simulink subsystem "A_LN_elliptical_inclined"  (R2022b)
settings: Solver=VariableStepAuto  StartTime=0.0  StopTime=10.0  RelTol=1e-3
undefined symbols (not defined in the file or in its folder): settings
libraries: matrix_library x1
settings Model: Creator=robertopistonenascone  LastModifiedBy=robertopistonenascone

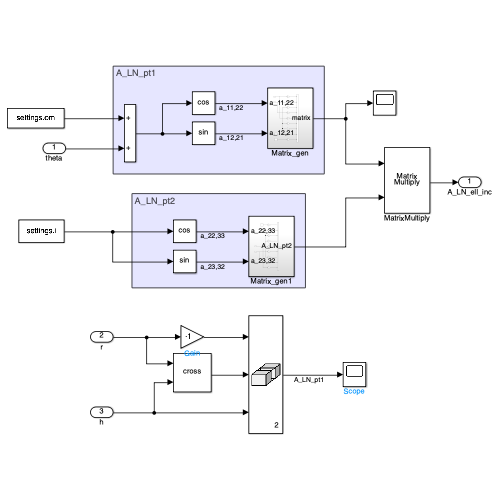
[thumbnail: Simulink's stored preview of the top-level diagram]
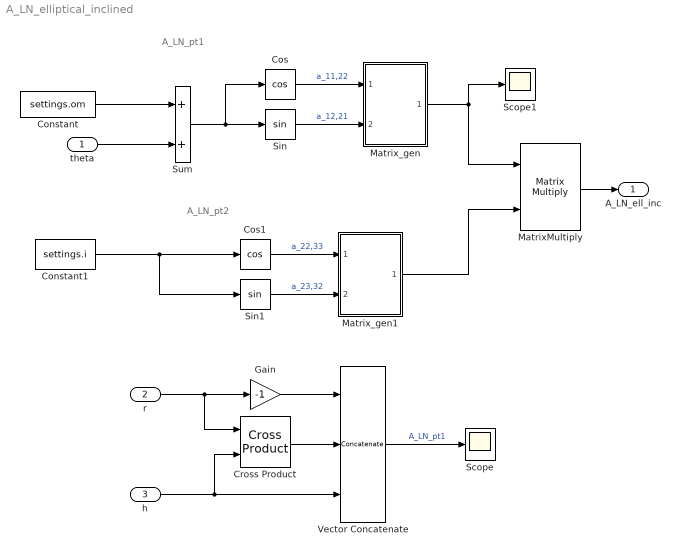
== system A_LN_elliptical_inclined ==
  note: A_LN_pt1
  note: A_LN_pt2
  theta : Inport
  r : Inport  Port=2
  h : Inport  Port=3
  Constant : Constant  Value=settings.om
  Constant1 : Constant  Value=settings.i
  Cos : Trigonometry  Operator=cos
  Cos1 : Trigonometry  Operator=cos
  Cross Product : matrix_library/Cross Product
  Gain : Gain  Gain=-1
  MatrixMultiply : Product  Multiplication=Matrix(*)
  Matrix_gen : Subsystem
  Matrix_gen1 : Subsystem
  Scope : Scope
  Scope1 : Scope
  Sin : Trigonometry
  Sin1 : Trigonometry
  Sum : Sum
  Vector Concatenate : Concatenate  NumInputs=3  Mode=Multidimensional array  ConcatenateDimension=2
  A_LN_ell_inc : Outport
  wires:
  MatrixMultiply/1 -> A_LN_ell_inc/1
  Matrix_gen/1(matrix) -> MatrixMultiply/1, Scope1/1
  Matrix_gen1/1(A_LN_pt2) -> MatrixMultiply/2
  Sum/1 -> Cos/1, Sin/1
  Cos1/1 -> Matrix_gen1/1(a_22,33)  "a_22,33"
  Constant1/1 -> Cos1/1, Sin1/1
  Cos/1 -> Matrix_gen/1(a_11,22)  "a_11,22"
  Sin/1 -> Matrix_gen/2(a_12,21)  "a_12,21"
  Constant/1 -> Sum/1
  Sin1/1 -> Matrix_gen1/2(a_23,32)  "a_23,32"
  theta/1 -> Sum/2
  Cross Product/1 -> Vector Concatenate/2
  r/1 -> Cross Product/1, Gain/1
  h/1 -> Cross Product/2, Vector Concatenate/3
  Vector Concatenate/1 -> Scope/1  "A_LN_pt1"
  Gain/1 -> Vector Concatenate/1

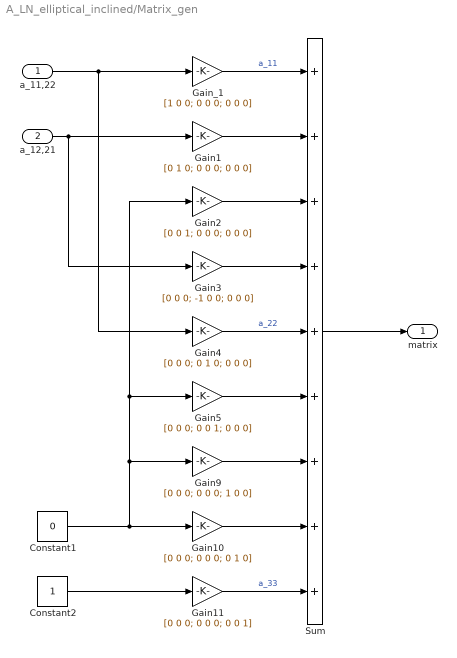
== system A_LN_elliptical_inclined/Matrix_gen ==
  a_11,22 : Inport
  a_12,21 : Inport  Port=2
  Constant1 : Constant  Value=0
  Constant2 : Constant
  Gain1 : Gain  Gain=[0 1 0; 0 0 0; 0 0 0]
  Gain10 : Gain  Gain=[0 0 0; 0 0 0; 0 1 0]
  Gain11 : Gain  Gain=[0 0 0; 0 0 0; 0 0 1]
  Gain2 : Gain  Gain=[0 0 1; 0 0 0; 0 0 0]
  Gain3 : Gain  Gain=[0 0 0; -1 0 0; 0 0 0]
  Gain4 : Gain  Gain=[0 0 0; 0 1 0; 0 0 0]
  Gain5 : Gain  Gain=[0 0 0; 0 0 1; 0 0 0]
  Gain9 : Gain  Gain=[0 0 0; 0 0 0; 1 0 0]
  Gain_1 : Gain  Gain=[1 0 0; 0 0 0; 0 0 0]
  Sum : Sum  Inputs=+++++++++
  matrix : Outport
  wires:
  Gain3/1 -> Sum/4
  Gain4/1 -> Sum/5  "a_22"
  Gain11/1 -> Sum/9  "a_33"
  Gain9/1 -> Sum/7
  a_12,21/1 -> Gain3/1, Gain1/1
  Gain_1/1 -> Sum/1  "a_11"
  Gain1/1 -> Sum/2
  Gain10/1 -> Sum/8
  Gain2/1 -> Sum/3
  Constant1/1 -> Gain2/1, Gain5/1, Gain9/1, Gain10/1
  a_11,22/1 -> Gain4/1, Gain_1/1
  Sum/1 -> matrix/1
  Constant2/1 -> Gain11/1
  Gain5/1 -> Sum/6

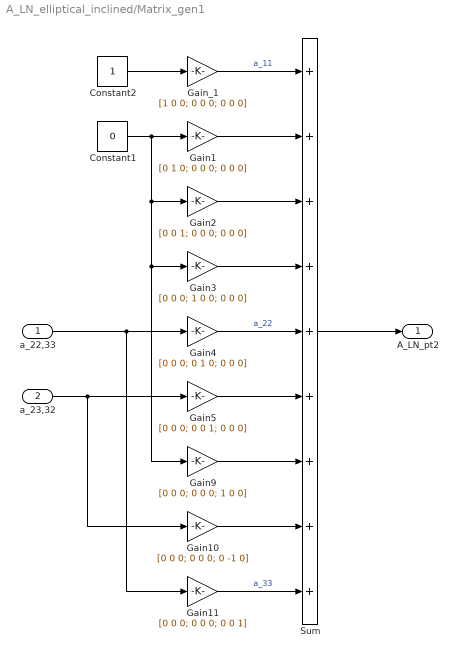
== system A_LN_elliptical_inclined/Matrix_gen1 ==
  a_22,33 : Inport
  a_23,32 : Inport  Port=2
  Constant1 : Constant  Value=0
  Constant2 : Constant
  Gain1 : Gain  Gain=[0 1 0; 0 0 0; 0 0 0]
  Gain10 : Gain  Gain=[0 0 0; 0 0 0; 0 -1 0]
  Gain11 : Gain  Gain=[0 0 0; 0 0 0; 0 0 1]
  Gain2 : Gain  Gain=[0 0 1; 0 0 0; 0 0 0]
  Gain3 : Gain  Gain=[0 0 0; 1 0 0; 0 0 0]
  Gain4 : Gain  Gain=[0 0 0; 0 1 0; 0 0 0]
  Gain5 : Gain  Gain=[0 0 0; 0 0 1; 0 0 0]
  Gain9 : Gain  Gain=[0 0 0; 0 0 0; 1 0 0]
  Gain_1 : Gain  Gain=[1 0 0; 0 0 0; 0 0 0]
  Sum : Sum  Inputs=+++++++++
  A_LN_pt2 : Outport
  wires:
  Gain3/1 -> Sum/4
  Gain4/1 -> Sum/5  "a_22"
  Gain11/1 -> Sum/9  "a_33"
  Gain9/1 -> Sum/7
  Gain_1/1 -> Sum/1  "a_11"
  Gain1/1 -> Sum/2
  Gain10/1 -> Sum/8
  Gain2/1 -> Sum/3
  Sum/1 -> A_LN_pt2/1
  Gain5/1 -> Sum/6
  Constant2/1 -> Gain_1/1
  Constant1/1 -> Gain2/1, Gain3/1, Gain9/1, Gain1/1
  a_22,33/1 -> Gain11/1, Gain4/1
  a_23,32/1 -> Gain5/1, Gain10/1
